simulink model "Decenteralized"  (R2025a)
settings: Solver=VariableStepAuto  StartTime=0.0  StopTime=10.0  RelTol=1e-3
undefined symbols (not defined in the file): DiscIntNeverNeededParam
libraries: ros2lib x3
settings Model: Creator=constanin  LastModifiedBy=constanin

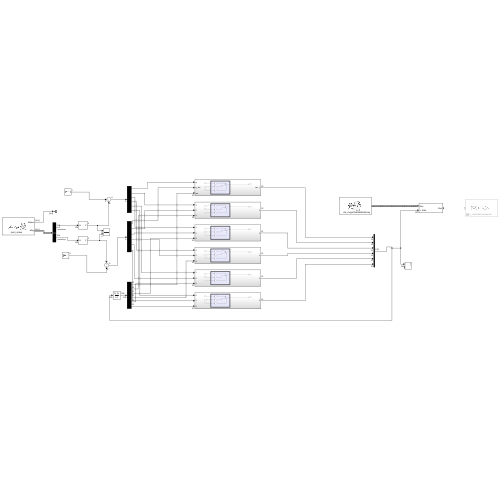
[thumbnail: Simulink's stored preview of the top-level diagram]
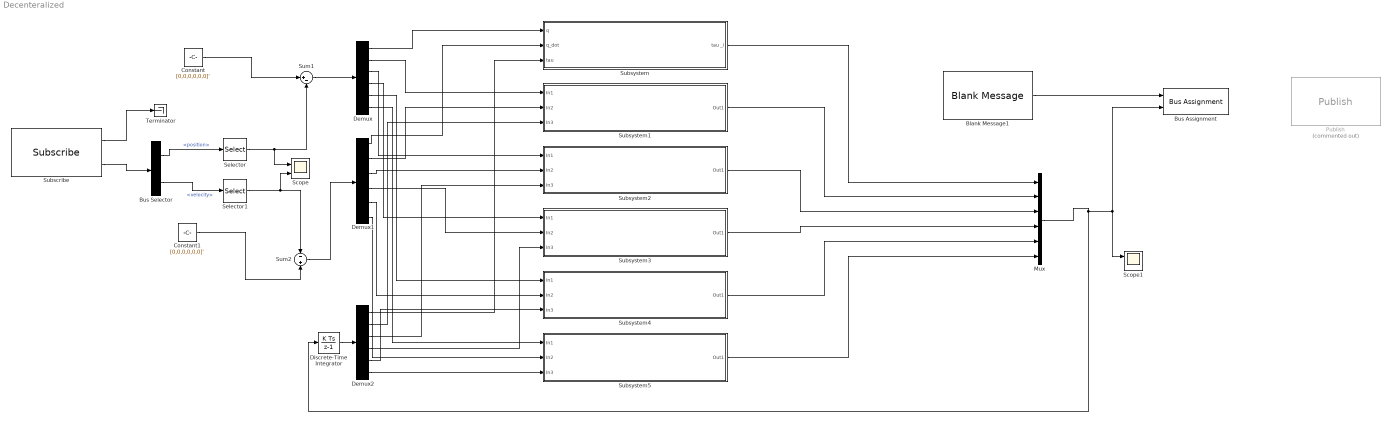
== system Decenteralized ==
  Blank Message1 : ros2lib/Blank Message  messageClass=Message  entityType=std_msgs/Float64MultiArray  messageType=std_msgs/Float64MultiArray  SampleTime=inf
  Bus Assignment : BusAssignment  AssignedSignals=data
  Bus Selector : BusSelector  OutputSignals=position,velocity
  Constant : Constant  Value=[0,0,0,0,0,0]'
  Constant1 : Constant  Value=[0,0,0,0,0,0]'
  Demux : Demux  Outputs=6
  Demux1 : Demux  Outputs=6
  Demux2 : Demux  Outputs=6
  Discrete-Time Integrator : DiscreteIntegrator  SampleTime=-1  ICPrevOutput=DiscIntNeverNeededParam  ICPrevScaledInput=DiscIntNeverNeededParam
  Mux : Mux  Inputs=6
  Publish : ros2lib/Publish  Commented=on  topicSource=Select from ROS network  topic=/forward_effort_controller/commands  messageType=std_msgs/Float64MultiArray  QOSHistory=Keep last  QOSDepth=10  QOSReliability=Reliable  QOSDurability=Volatile  QOSDeadline=Inf  QOSLifespan=Inf  QOSLiveliness=Automatic  QOSLeaseDuration=Inf  QOSAvoidROSNamespaceConventions=off
  Scope : Scope  NumInputPorts=2
      settings: ActiveDisplayYMinimum=-3.1817229992902876  ActiveDisplayYMaximum=1.6308390822232148  DataLoggingVariableName=ScopeData2  DataLoggingSaveFormat=Array
  Scope1 : Scope  NumInputPorts=2
      settings: ActiveDisplayYMinimum=-1  ActiveDisplayYMaximum=1  DataLoggingSaveFormat=Array
  Selector : Selector  InputPortWidth=128  IndexOptions=Index vector (dialog)  Indices=[1 2 3 4 5 6]  OutputSizes=1
  Selector1 : Selector  InputPortWidth=128  IndexOptions=Index vector (dialog)  Indices=[1 2 3 4 5 6]  OutputSizes=1
  Subscribe : ros2lib/Subscribe  topicSource=Select from ROS network  topic=/joint_states  messageType=sensor_msgs/JointState  sampleTime=-1  QOSHistory=Keep last  QOSDepth=10  QOSReliability=Reliable  QOSDurability=Volatile  QOSDeadline=Inf  QOSLifespan=Inf  QOSLiveliness=Automatic  QOSLeaseDuration=Inf  QOSAvoidROSNamespaceConventions=off
  Subsystem : Subsystem
  Subsystem1 : Subsystem
  Subsystem2 : Subsystem
  Subsystem3 : Subsystem
  Subsystem4 : Subsystem
  Subsystem5 : Subsystem
  Sum1 : Sum  Inputs=|+-
  Sum2 : Sum  Inputs=-|+
  Terminator : Terminator
  wires:
  Sum1/1 -> Demux/1
  Constant/1 -> Sum1/1
  Constant1/1 -> Sum2/2
  Sum2/1 -> Demux1/1
  Discrete-Time Integrator/1 -> Demux2/1
  Demux/1 -> Subsystem/1(q)
  Demux1/1 -> Subsystem/2(q_dot)
  Demux2/1 -> Subsystem/3(tau)
  Subsystem/1(tau _i) -> Mux/1
  Demux/2 -> Subsystem1/1(In1)
  Demux1/2 -> Subsystem1/2(In2)
  Demux2/2 -> Subsystem1/3(In3)
  Demux/3 -> Subsystem2/1(In1)
  Demux/4 -> Subsystem3/1(In1)
  Demux/5 -> Subsystem4/1(In1)
  Demux/6 -> Subsystem5/1(In1)
  Demux1/3 -> Subsystem2/2(In2)
  Demux1/4 -> Subsystem3/2(In2)
  Demux1/5 -> Subsystem4/2(In2)
  Demux1/6 -> Subsystem5/2(In2)
  Demux2/3 -> Subsystem2/3(In3)
  Demux2/4 -> Subsystem3/3(In3)
  Demux2/5 -> Subsystem4/3(In3)
  Demux2/6 -> Subsystem5/3(In3)
  Subscribe/2 -> Bus Selector/1
  Selector/1 -> Scope/1, Sum1/2
  Selector1/1 -> Scope/2, Sum2/1
  Subsystem1/1(Out1) -> Mux/2
  Subsystem2/1(Out1) -> Mux/3
  Subsystem3/1(Out1) -> Mux/4
  Subsystem4/1(Out1) -> Mux/5
  Subsystem5/1(Out1) -> Mux/6
  Blank Message1/1 -> Bus Assignment/1
  Mux/1 -> Scope1/1, Bus Assignment/2, Discrete-Time Integrator/1
  Bus Selector/1 -> Selector/1  "<position>"
  Bus Selector/2 -> Selector1/1  "<velocity>"
  Subscribe/1 -> Terminator/1

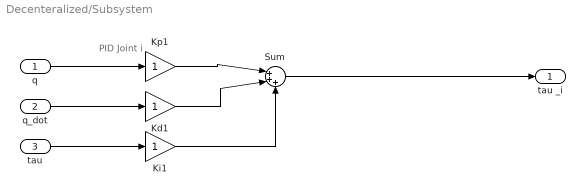
== system Decenteralized/Subsystem ==
  note: PID Joint i
  q : Inport
  q_dot : Inport  Port=2
  tau : Inport  Port=3
  Kd1 : Gain
  Ki1 : Gain
  Kp1 : Gain
  Sum : Sum  Inputs=|+++
  tau _i : Outport
  wires:
  q_dot/1 -> Kd1/1
  Kp1/1 -> Sum/1
  Kd1/1 -> Sum/2
  Ki1/1 -> Sum/3
  q/1 -> Kp1/1
  tau/1 -> Ki1/1
  Sum/1 -> tau _i/1

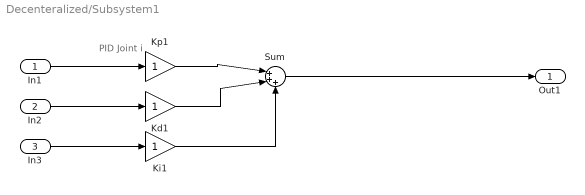
== system Decenteralized/Subsystem1 ==
  note: PID Joint i
  In1 : Inport
  In2 : Inport  Port=2
  In3 : Inport  Port=3
  Kd1 : Gain
  Ki1 : Gain
  Kp1 : Gain
  Sum : Sum  Inputs=|+++
  Out1 : Outport
  wires:
  In2/1 -> Kd1/1
  Kp1/1 -> Sum/1
  Kd1/1 -> Sum/2
  Ki1/1 -> Sum/3
  In1/1 -> Kp1/1
  In3/1 -> Ki1/1
  Sum/1 -> Out1/1

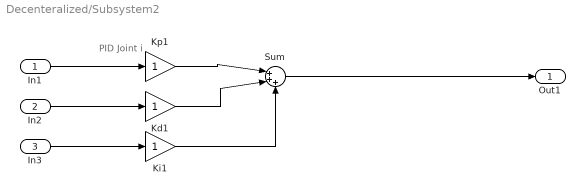
== system Decenteralized/Subsystem2 ==
  note: PID Joint i
  In1 : Inport
  In2 : Inport  Port=2
  In3 : Inport  Port=3
  Kd1 : Gain
  Ki1 : Gain
  Kp1 : Gain
  Sum : Sum  Inputs=|+++
  Out1 : Outport
  wires:
  In2/1 -> Kd1/1
  Kp1/1 -> Sum/1
  Kd1/1 -> Sum/2
  Ki1/1 -> Sum/3
  In1/1 -> Kp1/1
  In3/1 -> Ki1/1
  Sum/1 -> Out1/1

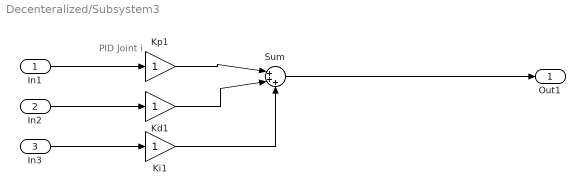
== system Decenteralized/Subsystem3 ==
  note: PID Joint i
  In1 : Inport
  In2 : Inport  Port=2
  In3 : Inport  Port=3
  Kd1 : Gain
  Ki1 : Gain
  Kp1 : Gain
  Sum : Sum  Inputs=|+++
  Out1 : Outport
  wires:
  In2/1 -> Kd1/1
  Kp1/1 -> Sum/1
  Kd1/1 -> Sum/2
  Ki1/1 -> Sum/3
  In1/1 -> Kp1/1
  In3/1 -> Ki1/1
  Sum/1 -> Out1/1

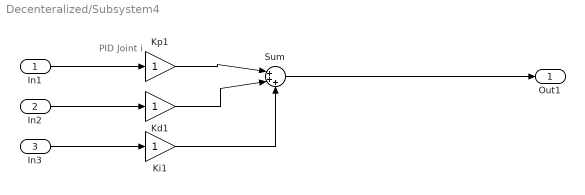
== system Decenteralized/Subsystem4 ==
  note: PID Joint i
  In1 : Inport
  In2 : Inport  Port=2
  In3 : Inport  Port=3
  Kd1 : Gain
  Ki1 : Gain
  Kp1 : Gain
  Sum : Sum  Inputs=|+++
  Out1 : Outport
  wires:
  In2/1 -> Kd1/1
  Kp1/1 -> Sum/1
  Kd1/1 -> Sum/2
  Ki1/1 -> Sum/3
  In1/1 -> Kp1/1
  In3/1 -> Ki1/1
  Sum/1 -> Out1/1

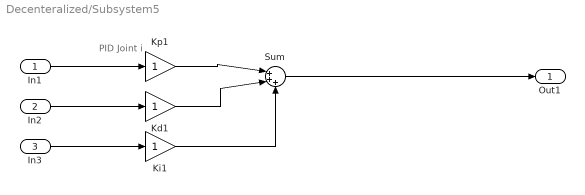
== system Decenteralized/Subsystem5 ==
  note: PID Joint i
  In1 : Inport
  In2 : Inport  Port=2
  In3 : Inport  Port=3
  Kd1 : Gain
  Ki1 : Gain
  Kp1 : Gain
  Sum : Sum  Inputs=|+++
  Out1 : Outport
  wires:
  In2/1 -> Kd1/1
  Kp1/1 -> Sum/1
  Kd1/1 -> Sum/2
  Ki1/1 -> Sum/3
  In1/1 -> Kp1/1
  In3/1 -> Ki1/1
  Sum/1 -> Out1/1
